simulink model "Energy_Flow_Model"  (R2023b)
settings: Solver=FixedStepAuto  StartTime=0.0  StopTime=1  FixedStep=2e-6  MaxStep=1e-5  RelTol=1e-3
values from neighbouring files (symbols this model uses):
  mems_b = b1+b2    (= 0.000950957529895)    [System_Analytics.m]
  mems_k = 2*((pi^4 / 6) * (E_silicon * t * w_s^3 / ((2*L_s1)^3+(2*L_s1)^3)))    (= 68.9981061491)    [System_Analytics.m]
  mems_mass = (calculate_proof_mass(length_m, width, thickness, density_si, N, comb_l,comb_w))    [System_Analytics.m]
libraries: fl_lib x21, nesl_utility x6, simulink x1
settings Model: Creator=241pr  LastModifiedBy=241pr
settings DataIOCC: SaveOutput=off  DSMLogging=off  SaveTime=off  ReturnWorkspaceOutputs=off

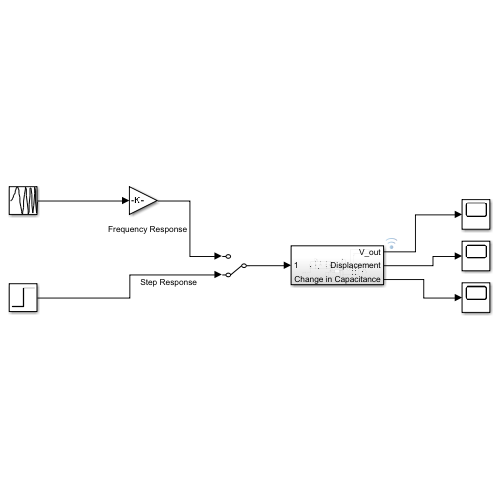
[thumbnail: Simulink's stored preview of the top-level diagram]
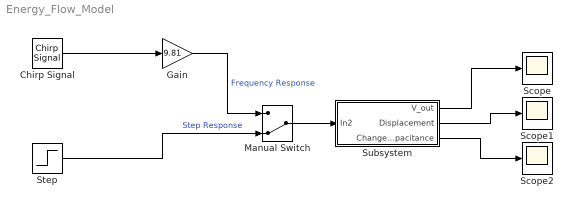
== system Energy_Flow_Model ==
  Chirp Signal : simulink/Sources/Chirp Signal  f1=1  T=1  f2=10000
  Gain : Gain  Gain=9.81
  Manual Switch : ManualSwitch  CurrentSetting=0
  Scope : Scope
  Scope1 : Scope
  Scope2 : Scope
  Step : Step  Time=0.2  After=9.81  SampleTime=1
  Subsystem : Subsystem
  wires:
  Subsystem/1(V_out) -> Scope/1
  Subsystem/2(Displacement) -> Scope1/1
  Subsystem/3(Change in Capacitance) -> Scope2/1
  Chirp Signal/1 -> Gain/1
  Manual Switch/1 -> Subsystem/1(In2)
  Gain/1 -> Manual Switch/1  "Frequency Response"
  Step/1 -> Manual Switch/2  "Step Response"

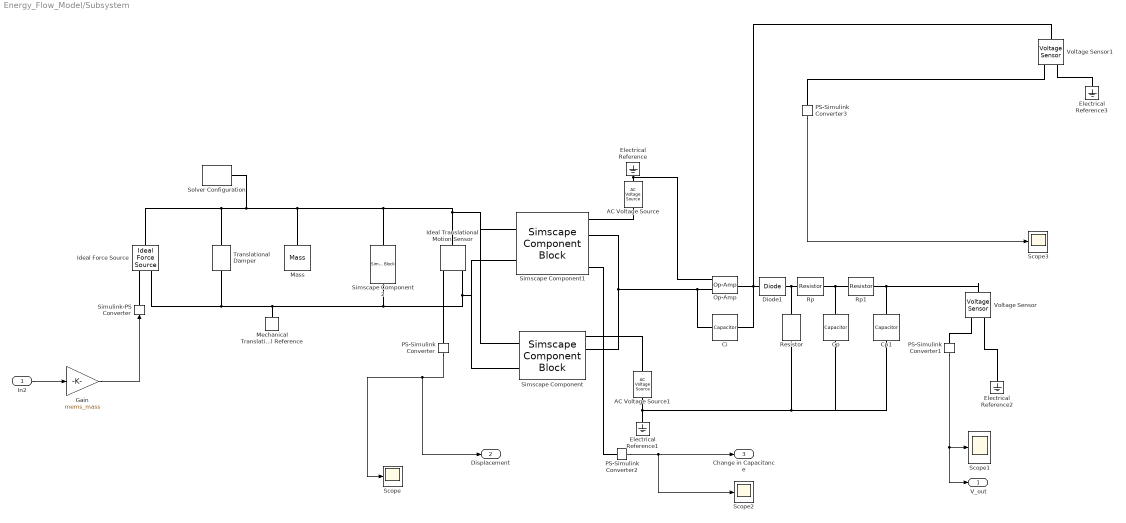
== system Energy_Flow_Model/Subsystem ==
  In2 : Inport
  AC Voltage Source : fl_lib/Electrical/Electrical Sources/AC Voltage Source  amp=5 V  shift=0 deg  frequency=5e4 Hz  omega=0 rad/s
  AC Voltage Source1 : fl_lib/Electrical/Electrical Sources/AC Voltage Source  amp=5 V  shift=180 deg  frequency=5e4 Hz  omega=0 rad/s
  Ci : fl_lib/Electrical/Electrical Elements/Capacitor  c=3.45e-13 F  r=1e-6 Ohm  g=0 1/Ohm  i_specify=off  i_priority=None  i=0 A  i_nominal_specify=off  i_nominal_unit=A  i_nominal_value=1  v_specify=off  v_priority=None  v=0 V  v_nominal_specify=off  v_nominal_unit=V  v_nominal_value=1  vc_specify=off  vc_priority=High  vc=0 V  vc_nominal_specify=off  vc_nominal_unit=V  vc_nominal_value=1
  Cp : fl_lib/Electrical/Electrical Elements/Capacitor  c=16 nF  r=1e-6 Ohm  g=0 1/Ohm  i_specify=off  i_priority=None  i=0 A  i_nominal_specify=off  i_nominal_unit=A  i_nominal_value=1  v_specify=off  v_priority=None  v=0 V  v_nominal_specify=off  v_nominal_unit=V  v_nominal_value=1  vc_specify=off  vc_priority=High  vc=0 V  vc_nominal_specify=off  vc_nominal_unit=V  vc_nominal_value=1
  Cp1 : fl_lib/Electrical/Electrical Elements/Capacitor  c=16 nF  r=1e-6 Ohm  g=0 1/Ohm  i_specify=off  i_priority=None  i=0 A  i_nominal_specify=off  i_nominal_unit=A  i_nominal_value=1  v_specify=off  v_priority=None  v=0 V  v_nominal_specify=off  v_nominal_unit=V  v_nominal_value=1  vc_specify=off  vc_priority=High  vc=0 V  vc_nominal_specify=off  vc_nominal_unit=V  vc_nominal_value=1
  Diode1 : fl_lib/Electrical/Electrical Elements/Diode  Vf=0.09 V  Ron=0.3 Ohm  Goff=1e-8 1/Ohm  i_specify=off  i_priority=None  i=0 A  i_nominal_specify=off  i_nominal_unit=A  i_nominal_value=1  v_specify=off  v_priority=None  v=0 V  v_nominal_specify=off  v_nominal_unit=V  v_nominal_value=1
  Electrical Reference{,1..3} (4 alike) : fl_lib/Electrical/Electrical Elements/Electrical Reference
  Gain : Gain  Gain=mems_mass
  Ideal Force Source : fl_lib/Mechanical/Mechanical Sources/Ideal Force Source
  Ideal Translational Motion Sensor : fl_lib/Mechanical/Mechanical Sensors/Ideal Translational Motion Sensor  reference=foundation.enum.MeasurementReference.difference  acceleration_port=false  velocity_port=true  position_port=true  offset=0 m
  Mass : fl_lib/Mechanical/Translational Elements/Mass  mass=mems_mass kg  num_ports=foundation.enum.numPorts2.one  v_specify=off  v_priority=High  v=0 m/s  v_nominal_specify=off  v_nominal_unit=m/s  v_nominal_value=1  f_specify=off  f_priority=None  f=0 N  f_nominal_specify=off  f_nominal_unit=N  f_nominal_value=1
  Mechanical Translational Reference : fl_lib/Mechanical/Translational Elements/Mechanical Translational Reference
  Op-Amp : fl_lib/Electrical/Electrical Elements/Op-Amp  outI_specify=off  outI_priority=None  outI=0 A  outI_nominal_specify=off  outI_nominal_unit=A  outI_nominal_value=1
  PS-Simulink Converter{,1..3} (4 alike) : nesl_utility/PS-Simulink Converter  PhysicalDomain=network_engine_domain  SubClassName=ps_output  LeftPortType=input  RightPortType=output  PseudoPeriodic=off  Frequencies=[]  VectorFormat=inherit  Unit=inherit  AffineConversion=off
  Resistor : fl_lib/Electrical/Electrical Elements/Resistor  R=1e6 Ohm  i_specify=off  i_priority=None  i=0 A  i_nominal_specify=off  i_nominal_unit=A  i_nominal_value=1  v_specify=off  v_priority=None  v=0 V  v_nominal_specify=off  v_nominal_unit=V  v_nominal_value=1
  Rp : fl_lib/Electrical/Electrical Elements/Resistor  R=1e4 Ohm  i_specify=off  i_priority=None  i=0 A  i_nominal_specify=off  i_nominal_unit=A  i_nominal_value=1  v_specify=off  v_priority=None  v=0 V  v_nominal_specify=off  v_nominal_unit=V  v_nominal_value=1
  Rp1 : fl_lib/Electrical/Electrical Elements/Resistor  R=1e4 Ohm  i_specify=off  i_priority=None  i=0 A  i_nominal_specify=off  i_nominal_unit=A  i_nominal_value=1  v_specify=off  v_priority=None  v=0 V  v_nominal_specify=off  v_nominal_unit=V  v_nominal_value=1
  Scope{,1..3} (4 alike) : Scope
  Simscape Component : SimscapeComponentBlock  SourceFile=EMdiport_GV_neg  ComponentPath=EMdiport_GV_neg  ComponentVariants="[\"EMdiport_GV_neg\"]"  ComponentVariantNames="[\"EMdiport_GV_neg\"]"  ClassName=EMdiport_GV_neg  SchemaVersion=1  Co=C1 F  do=d1 m  u_specify=off  u_priority=None  u=0 V  u_nominal_specify=off  u_nominal_unit=V  u_nominal_value=1  i_specify=off  i_priority=None  i=0 A  i_nominal_specify=off  i_nominal_unit=A  i_nominal_value=1  v_specify=off  v_priority=None  v=0 m/s  v_nominal_specify=off  v_nominal_unit=m/s  v_nominal_value=1  f_specify=off  f_priority=None  f=0 N  f_nominal_specify=off  f_nominal_unit=N  f_nominal_value=1  x_specify=off  x_priority=None  x=0 m  x_nominal_specify=off  x_nominal_unit=m  x_nominal_value=1  del_C_specify=off  del_C_priority=None  del_C=0 F/m  del_C_nominal_specify=off  del_C_nominal_unit=F/m  del_C_nominal_value=1
      settings: CopyFcn=simscape.engine.sli.internal.componentblockcallback(gcbh,'COPY')  PreCopyFcn=simscape.engine.sli.internal.componentblockcallback(gcbh,'PRECOPY')  PreDeleteFcn=simscape.engine.sli.internal.componentblockcallback(gcbh,'PREDELETE')  InternalSimscapePortConfiguration="{\"Bottom\":[],\"Left\":[{\"id\":\"pm\",\"label\":\"m+\",\"type\":\"foundation.mechanical.translational.translational\"},{\"id\":\"nm\",\"label\":\"m-\",\"type\":\"foundation.mechanical.translational.translational\"}],\"Right\":[{\"id\":\"pe\",\"label\":\"e+\",\"type\":\"foundation.electrical.electrical\"},{\"id\":\"ne\",\"label\":\"e-\",\"type\":\"foundation.electrical.electrical\"},{\"id\":\"dc\",\"label\":\"dc\",\"type\":\"output\"},{\"id\":\"C\",\"label\":\"C(t)\",\"type\":\"output\"}],\"Top\":[]}"
      mask Type: EMdiport_GV_neg
  Simscape Component1 : SimscapeComponentBlock  SourceFile=EMdiport_GV_pos  ComponentPath=EMdiport_GV_pos  ComponentVariants="[\"EMdiport_GV_pos\"]"  ComponentVariantNames="[\"EMdiport_GV_pos\"]"  ClassName=EMdiport_GV_pos  SchemaVersion=1  Co=C1 F  do=d1 m  u_specify=off  u_priority=None  u=0 V  u_nominal_specify=off  u_nominal_unit=V  u_nominal_value=1  i_specify=off  i_priority=None  i=0 A  i_nominal_specify=off  i_nominal_unit=A  i_nominal_value=1  v_specify=off  v_priority=None  v=0 m/s  v_nominal_specify=off  v_nominal_unit=m/s  v_nominal_value=1  f_specify=off  f_priority=None  f=0 N  f_nominal_specify=off  f_nominal_unit=N  f_nominal_value=1  x_specify=off  x_priority=None  x=0 m  x_nominal_specify=off  x_nominal_unit=m  x_nominal_value=1  del_C_specify=off  del_C_priority=None  del_C=0 F/m  del_C_nominal_specify=off  del_C_nominal_unit=F/m  del_C_nominal_value=1
      settings: CopyFcn=simscape.engine.sli.internal.componentblockcallback(gcbh,'COPY')  PreCopyFcn=simscape.engine.sli.internal.componentblockcallback(gcbh,'PRECOPY')  PreDeleteFcn=simscape.engine.sli.internal.componentblockcallback(gcbh,'PREDELETE')  InternalSimscapePortConfiguration="{\"Bottom\":[],\"Left\":[{\"id\":\"pm\",\"label\":\"m+\",\"type\":\"foundation.mechanical.translational.translational\"},{\"id\":\"nm\",\"label\":\"m-\",\"type\":\"foundation.mechanical.translational.translational\"}],\"Right\":[{\"id\":\"pe\",\"label\":\"e+\",\"type\":\"foundation.electrical.electrical\"},{\"id\":\"ne\",\"label\":\"e-\",\"type\":\"foundation.electrical.electrical\"},{\"id\":\"dc\",\"label\":\"dc\",\"type\":\"output\"},{\"id\":\"C\",\"label\":\"C(t)\",\"type\":\"output\"}],\"Top\":[]}"
      mask Type: EMdiport_GV_pos
  Simscape Component2 : SimscapeComponentBlock  SourceFile=nonlinear_spring  ComponentPath=nonlinear_spring  ComponentVariants="[\"nonlinear_spring\"]"  ComponentVariantNames="[\"nonlinear_spring\"]"  ClassName=nonlinear_spring  SchemaVersion=1  k=mems_k N/m  dstop=10 um  v_specify=off  v_priority=None  v=0 m/s  v_nominal_specify=off  v_nominal_unit=m/s  v_nominal_value=1  f_specify=off  f_priority=None  f=0 N  f_nominal_specify=off  f_nominal_unit=N  f_nominal_value=1  x_specify=off  x_priority=High  x=0 m  x_nominal_specify=off  x_nominal_unit=m  x_nominal_value=1
      settings: CopyFcn=simscape.engine.sli.internal.componentblockcallback(gcbh,'COPY')  PreCopyFcn=simscape.engine.sli.internal.componentblockcallback(gcbh,'PRECOPY')  PreDeleteFcn=simscape.engine.sli.internal.componentblockcallback(gcbh,'PREDELETE')  InternalSimscapePortConfiguration="{\"Bottom\":[],\"Left\":[{\"id\":\"R\",\"label\":\"R\",\"type\":\"foundation.mechanical.translational.translational\"}],\"Right\":[{\"id\":\"C\",\"label\":\"C\",\"type\":\"foundation.mechanical.translational.translational\"}],\"Top\":[]}"
      mask Type: nonlinear_spring
  Simulink-PS Converter : nesl_utility/Simulink-PS Converter  PhysicalDomain=network_engine_domain  SubClassName=ps_input  LeftPortType=input  RightPortType=output  PseudoPeriodic=off  Frequencies=[]  NoiseDistribution=none  NoiseParameters=[]  Unit=1  AffineConversion=off  FilteringAndDerivatives=provide  SimscapeFilterOrder=1  InputFilterTimeConstant=0.001  UdotUserProvided=0
  Solver Configuration : nesl_utility/Solver Configuration  PhysicalDomain=network_engine_domain  SubClassName=solver  LeftPortType=input  RightPortType=generic  Tones=[]  Harmonics=[]  SimulateNoise=off  Profile=off  UseLocalSampling=off  EnableSwitchedLinearOptims=on  FrequencyDomain=off  UseCCode=off  RelTol=0.001  AbsTol=0.001  MinStep=1e-09  ToWorkspace=off  RevertToSquareIcSolve=off  NumHomotopyIterations=100  PhasorMode=off  PhasorModeNumHarmonics=1  ConsistencySolver=NEWTON_XTOL_AFTER_FTOL  IndexReductionMethod=DerivativeReplacement  DoDC=off  ResidualTolerance=1e-09  ConsistencyTolSource=GLOBAL  ConsistencyAbsTol=0.001  ConsistencyRelTol=0.001  ConsistencyTolFactor=0.001  UseLocalSolver=on  LocalSolverChoice=NE_BACKWARD_EULER_ADVANCER  ResolveIndetEquations=on  FunctionEvalNumThread=1  LocalSolverSampleTime=2e-6  DoFixedCost=on  MaxNonlinIter=3  MaxModeIter=2  ComputeImpulses=off  ImpulseIterations=2  LinearAlgebra=auto  LinearAlgebraNumThread=0  EquationFormulation=NE_TIME_EF  DelaysMemoryBudget=1024  AutomaticFiltering=on  FilteringTimeConstant=0.001  PartitionStorageMethod=AS_NEEDED  PartitionMemoryBudget=1024  PartitionMethod=ROBUST  MultibodyUseLocalSolver=off  MultibodyLocalSolverChoice=ODE1  MultibodyLocalSolverSampleTime=0.001
  Translational Damper : fl_lib/Mechanical/Translational Elements/Translational Damper  D=mems_b N*s/m  v_specify=off  v_priority=None  v=0 m/s  v_nominal_specify=off  v_nominal_unit=m/s  v_nominal_value=1  f_specify=off  f_priority=None  f=0 N  f_nominal_specify=off  f_nominal_unit=N  f_nominal_value=1
  Voltage Sensor : fl_lib/Electrical/Electrical Sensors/Voltage Sensor
  Voltage Sensor1 : fl_lib/Electrical/Electrical Sensors/Voltage Sensor
  V_out : Outport
  Displacement : Outport  Port=2
  Change in Capacitance : Outport  Port=3
  wires:
  Gain/1 -> Simulink-PS Converter/1
  PS-Simulink Converter/1 -> Displacement/1, Scope/1
  PS-Simulink Converter1/1 -> Scope1/1, V_out/1
  PS-Simulink Converter2/1 -> Scope2/1, Change in Capacitance/1
  In2/1 -> Gain/1
  PS-Simulink Converter3/1 -> Scope3/1
  connections:
  Simulink-PS Converter/RConn1 -- Ideal Force Source/RConn1
  Ideal Force Source/LConn1 -- Translational Damper/LConn1 -- Solver Configuration/RConn1 -- Mass/LConn1 -- Simscape Component2/LConn1 -- Simscape Component1/LConn1 -- Simscape Component/LConn1 -- Ideal Translational Motion Sensor/LConn1
  Ideal Force Source/RConn2 -- Translational Damper/RConn1 -- Mechanical Translational Reference/LConn1 -- Simscape Component2/RConn1 -- Simscape Component1/LConn2 -- Simscape Component/LConn2 -- Ideal Translational Motion Sensor/RConn1
  PS-Simulink Converter/LConn1 -- Ideal Translational Motion Sensor/RConn3
  AC Voltage Source/LConn1 -- Simscape Component1/RConn1
  Electrical Reference/LConn1 -- Op-Amp/LConn1 -- AC Voltage Source/RConn1
  Electrical Reference1/LConn1 -- Cp1/RConn1 -- Cp/RConn1 -- Resistor/RConn1 -- AC Voltage Source1/RConn1
  Ci/LConn1 -- Op-Amp/LConn2 -- Simscape Component/RConn2 -- Simscape Component1/RConn2
  Ci/RConn1 -- Diode1/LConn1 -- Op-Amp/RConn1 -- Voltage Sensor1/LConn1
  Rp/RConn1 -- Rp1/LConn1 -- Cp/LConn1
  Voltage Sensor/RConn1 -- PS-Simulink Converter1/LConn1
  Rp/LConn1 -- Resistor/LConn1 -- Diode1/RConn1
  Simscape Component/RConn1 -- AC Voltage Source1/LConn1
  Electrical Reference2/LConn1 -- Voltage Sensor/RConn2
  Simscape Component1/RConn4 -- PS-Simulink Converter2/LConn1
  Electrical Reference3/LConn1 -- Voltage Sensor1/RConn2
  Voltage Sensor1/RConn1 -- PS-Simulink Converter3/LConn1
  Rp1/RConn1 -- Voltage Sensor/LConn1 -- Cp1/LConn1
